simulink model "racecarMPCsim"  (R2018b)
settings: Solver=FixedStepAuto  StartTime=0.0  StopTime=7.6  FixedStep=0.1  RelTol=1e-3
libraries: simulink x2, mpclib x1
settings Model: Creator=reiserbalazs  LastModifiedBy=reiserbalazs

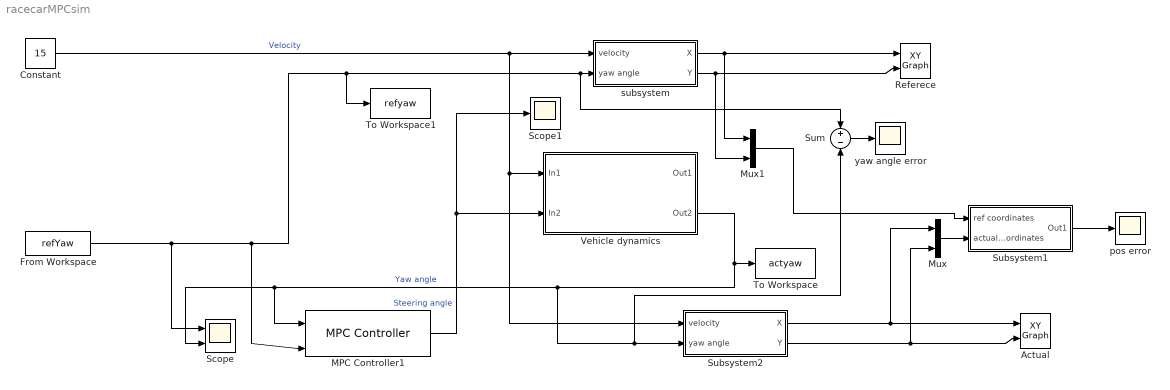
== system racecarMPCsim ==
  Actual : simulink/Sinks/XY Graph  xmin=-20  xmax=80  ymin=-80  ymax=80  st=-1
  Constant : Constant  Value=15
  From Workspace : FromWorkspace  VariableName=refYaw  SampleTime=0
  MPC Controller1 : mpclib/MPC Controller  SCDEnableBlockLinearizationSpecification=on  mpcobj=mpc1  is_multiple=0  enable_value=0  return_u0=off  updateMPCinCallerWorkspace=on  md_inport=off  mv_inport=off  return_cost=off  return_mvseq=off  return_qpstatus=off  return_xseq=off  return_state=off  return_ovseq=off  state_inport=off  umin_inport=off  umax_inport=off  ymin_inport=off  ymax_inport=off  cc_inport=off  ywt_inport=off  uwt_inport=off  duwt_inport=off  rhoeps_inport=off  uref_inport=off  n_ts=0.1  n_p=10  n_mv=1  n_md=0  n_ud=0  n_mo=1  n_uo=0  BlockDataType=double  SampleTimeInherited=off  switch_inport=off
  Mux : Mux  Inputs=2
  Mux1 : Mux  Inputs=2
  Referece : simulink/Sinks/XY Graph  xmin=-20  xmax=80  ymin=-80  ymax=60  st=-1
  Scope : Scope  NumInputPorts=2
  Scope1 : Scope
  Subsystem1 : Subsystem
  Subsystem2 : Subsystem
  Sum : Sum  Inputs=+-
  To Workspace : ToWorkspace  VariableName=actyaw  SaveFormat=Timeseries  SampleTime=-1
  To Workspace1 : ToWorkspace  VariableName=refyaw  SaveFormat=Timeseries  SampleTime=-1
  Vehicle dynamics : Subsystem
      mask Display: image('formulacargray.png');
  pos error : Scope
  "subsystem " : Subsystem
  yaw angle error : Scope
  wires:
  Constant/1 -> "subsystem "/1(velocity), Subsystem2/1(velocity), Vehicle dynamics/1(In1)  "Velocity"
  Vehicle dynamics/2(Out2) -> To Workspace/1, Sum/2, Subsystem2/2(yaw angle), MPC Controller1/1, Scope/2  "Yaw angle"
  From Workspace/1 -> Scope/1, MPC Controller1/2, To Workspace1/1, Sum/1, "subsystem "/2(yaw angle)
  "subsystem "/1(X) -> Mux1/1, Referece/1
  "subsystem "/2(Y) -> Referece/2, Mux1/2
  Subsystem2/1(X) -> Mux/1, Actual/1
  Subsystem2/2(Y) -> Mux/2, Actual/2
  MPC Controller1/1 -> Vehicle dynamics/2(In2), Scope1/1  "Steering angle"
  Sum/1 -> yaw angle error/1
  Mux/1 -> Subsystem1/2(actual coordinates)
  Mux1/1 -> Subsystem1/1(ref coordinates)
  Subsystem1/1(Out1) -> pos error/1

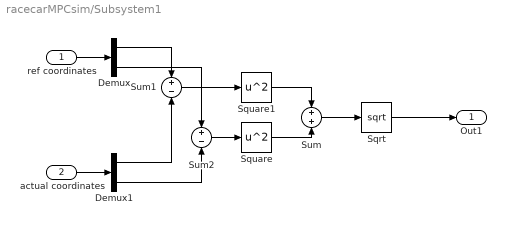
== system racecarMPCsim/Subsystem1 ==
  ref coordinates : Inport
  actual coordinates : Inport  Port=2
  Demux : Demux  Outputs=2
  Demux1 : Demux  Outputs=2
  Sqrt : Sqrt  SaturateOnIntegerOverflow=on
  Square : Math  Operator=square  SaturateOnIntegerOverflow=on
  Square1 : Math  Operator=square  SaturateOnIntegerOverflow=on
  Sum : Sum
  Sum1 : Sum  Inputs=+-
  Sum2 : Sum  Inputs=+-
  Out1 : Outport
  wires:
  ref coordinates/1 -> Demux/1
  actual coordinates/1 -> Demux1/1
  Demux/1 -> Sum1/1
  Demux1/1 -> Sum1/2
  Demux/2 -> Sum2/1
  Demux1/2 -> Sum2/2
  Sum1/1 -> Square1/1
  Sum2/1 -> Square/1
  Square1/1 -> Sum/1
  Square/1 -> Sum/2
  Sum/1 -> Sqrt/1
  Sqrt/1 -> Out1/1

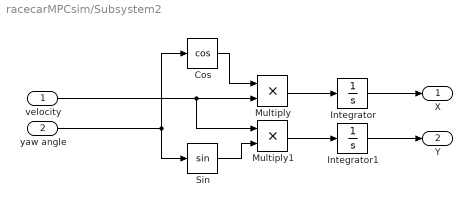
== system racecarMPCsim/Subsystem2 ==
  velocity : Inport
  yaw angle : Inport  Port=2
  Cos : Trigonometry  Operator=cos
  Integrator : Integrator
  Integrator1 : Integrator
  Multiply : Product
  Multiply1 : Product
  Sin : Trigonometry
  X : Outport
  Y : Outport  Port=2
  wires:
  velocity/1 -> Multiply/2, Multiply1/1
  Cos/1 -> Multiply/1
  Sin/1 -> Multiply1/2
  yaw angle/1 -> Sin/1, Cos/1
  Multiply/1 -> Integrator/1
  Multiply1/1 -> Integrator1/1
  Integrator/1 -> X/1
  Integrator1/1 -> Y/1

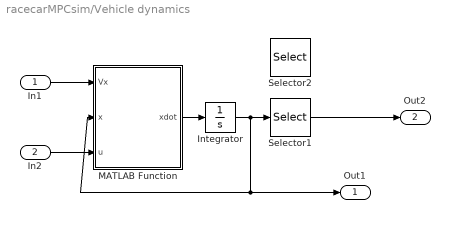
== system racecarMPCsim/Vehicle dynamics ==
  In1 : Inport
  In2 : Inport  Port=2
  Integrator : Integrator
  MATLAB Function : MATLAB Function  TreatAsAtomicUnit=on
  Selector1 : Selector  InputPortWidth=4  IndexOptions=Index vector (dialog)  Indices=3  OutputSizes=1
  Selector2 : Selector  InputPortWidth=4  IndexOptions=Index vector (dialog)  Indices=3  OutputSizes=1
  Out1 : Outport
  Out2 : Outport  Port=2
  wires:
  MATLAB Function/1(xdot) -> Integrator/1
  Integrator/1 -> Out1/1, MATLAB Function/2(x), Selector1/1
  In1/1 -> MATLAB Function/1(Vx)
  In2/1 -> MATLAB Function/3(u)
  Selector1/1 -> Out2/1

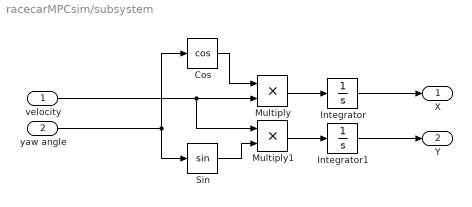
== system racecarMPCsim/subsystem  ==
  velocity : Inport
  yaw angle : Inport  Port=2
  Cos : Trigonometry  Operator=cos
  Integrator : Integrator
  Integrator1 : Integrator
  Multiply : Product
  Multiply1 : Product
  Sin : Trigonometry
  X : Outport
  Y : Outport  Port=2
  wires:
  Multiply/1 -> Integrator/1
  Multiply1/1 -> Integrator1/1
  velocity/1 -> Multiply/2, Multiply1/1
  Cos/1 -> Multiply/1
  Sin/1 -> Multiply1/2
  yaw angle/1 -> Sin/1, Cos/1
  Integrator/1 -> X/1
  Integrator1/1 -> Y/1

== matlab function racecarMPCsim/Vehicle dynamics/MATLAB Function ==
  data: Vx input; x input size=[4,1]; u input; xdot output size=[4,1]
function xdot = fcn(Vx,x,u)

% Model parameters
% m = 293;
% lw = 1.4;
% Ltotal = 2.3;
% Iz = m*(lw^2 + Ltotal^2)/12;
% lf = 0.85;
% lr = 0.75;
% Cf = 12000;
% Cr = 20000;

m = 1575;
Iz = 2875;
lf = 1.2;
lr = 1.6;
Cf = 19000;
Cr = 33000;

% Continuous-time model
A = [-(2*Cf+2*Cr)/m/Vx, 0, -Vx-(2*Cf*lf-2*Cr*lr)/m/Vx, 0;
     0, 0, 1, 0;
     -(2*Cf*lf-2*Cr*lr)/Iz/Vx, 0, -(2*Cf*lf^2+2*Cr*lr^2)/Iz/Vx, 0;
     1, Vx, 0, 0];
B = [2*Cf/m 0 2*Cf*lf/Iz 0]';
C = [0 0 0 1; 0 1 0 0];
D = zeros(2,1);
xdot = A*x + B*u;
%y = C*x + D*u;
